simulink library "myLibrary"  (R2023b)
settings: Solver=VariableStepAuto  StartTime=0.0  StopTime=10.0  RelTol=1e-3
undefined symbols (not defined in the file): Cac_n1, ctrl1, Da, delta_slk, Discrete, dtha, ee_sli_rtmsupport, FA, gcbh, Ha, Ini, init_DCline, init_IPC, init_line, init_load, init_SG, init_shunt, init_TH, init_trafo, init_user, init_VSC, initMachineBlocks, Ka, Lf, Llkd_pu, Llkq1_pu, magnitude, NET, P, plots_step, q0, Rac_n1, Radd, Rkd_pu, Rkq1_pu, Rload_add, sim_config, sps_rtmsupport, spsSteamTurbineModel, T_DC_NET, T_global, T_IPC, T_load, T_NET, T_SG, T_shunt, T_STATCOM, T_TH, T_trafo, T_user, T_VSC, Ts, tstep, Udiff_a, V1
libraries: spsSeriesRLCBranchLib x120, eeGeneralControl x83, $bdroot x78, spsCurrentMeasurementLib x53, spsParallelRLCBranchLib x39, spsVoltageMeasurementLib x37, spsControlledVoltageSourceLib x30, simulink x29, spsFirstOrderFilterLib x18, spsMeasurementModel x13, spsThreePhaseVIMeasurementLib x5, dspsigops x4
(part 5 of 16)

== system myLibrary/WT ==
  Constant1 : Constant  Value=[ 2/3 1/3; -1/3 1/3 ; -1/3 -2/3]
  Constant5 : Constant  Value=[ 2/3 1/3; -1/3 1/3 ; -1/3 -2/3]
  Control : Subsystem
      settings: PortSchema="{\"entries\":[{\"content\":{\"sides\":[{\"content\":{},\"type\":\"ConnectorPlacement.EquallySpacedRectSide\",\"uuid\":\"681c0b5f-022d-4b6d-8fe2-73940743a76e\"},{\"content\":{\"side\":\"RIGHT\"},\"type\":\"ConnectorPlacement.EquallySpacedRectSide\",\"uuid\":\"e9b400c8-e13f-4caf-91a1-f348979675fd\"},{\"content\":{\"connectorIds\":[\"In1\",\"Out1\",\"Out2\"],\"side\":\"TOP\"},\"type\":\"ConnectorPlacement.EquallySpacedRectSide\",\"uuid\":\"348007cb-ce67-4c45-ad7b-36ba89db6185\"},{\"content\":{\"connectorIds\":[\"In2\",\"In3\",\"In4\",\"In5\"],\"side\":\"BOTTOM\"},\"type\":\"ConnectorPlacement.EquallySpacedRectSide\",\"uuid\":\"fd6a847a-5d69-44cd-a0d1-495126761350\"}]},\"type\":\"ConnectorPlacement.EquallySpacedConnector\",\"uuid\":\"d16b8cae-5ced-4c76-a87e-983e154fb48f\"}],\"packageUris\":[\"http://schema.mathworks.com/mf0/Connector/R2020b\"],\"version\":\"1.0\"}"
  Current Measurement20 : spsCurrentMeasurementLib/Current Measurement  PhasorSimulation=off  OutputType=Complex  PSBequivalent=0
  Current Measurement21 : spsCurrentMeasurementLib/Current Measurement  PhasorSimulation=off  OutputType=Complex  PSBequivalent=0
  Current Measurement25 : spsCurrentMeasurementLib/Current Measurement  PhasorSimulation=off  OutputType=Complex  PSBequivalent=0
  Delay : Subsystem
  Electrical : Subsystem
  Filter Ig : Subsystem
  Filter Is : Subsystem
  Filter U : Subsystem
  Filter Vdc : Subsystem
  Filter Vg : Subsystem
  Gain : Gain  Gain=sqrt(2)/sqrt(3)
  Ig_l2g : Gain  Gain=1/T_VSC.Sbpu_l2g
  Ig_l2g1 : Gain  Gain=sqrt(3/2)
  Ig_l2g2 : Gain  Gain=sqrt(3/2)
  Is_l2g : Gain  Gain=1/T_VSC.Sbpu_l2g
  Mux1 : Mux  Inputs=2
  Mux10 : Mux  Inputs=2
  Mux4 : Mux  Inputs=3
  Product1 : Product  Multiplication=Matrix(*)
  Product4 : Product  Multiplication=Matrix(*)
  Series RLC Branch1 : spsSeriesRLCBranchLib/Series RLC Branch  LConnTagsString=__new0  RConnTagsString=__new0  BranchType=RL  Resistance=initVSC.Rtr  Inductance=initVSC.Ltr  SetiL0=off  InitialCurrent=initVSC.Iga  Capacitance=P.C  Setx0=on  InitialVoltage=P.C  Measurements=None
  Series RLC Branch10 : spsSeriesRLCBranchLib/Series RLC Branch  LConnTagsString=__new0  RConnTagsString=__new0  BranchType=R  Resistance=initVSC.Rac  Inductance=Lf  SetiL0=off  InitialCurrent=0  Capacitance=Cac_n1  Setx0=on  InitialVoltage=vcini_n1  Measurements=None
  Series RLC Branch2 : spsSeriesRLCBranchLib/Series RLC Branch  LConnTagsString=__new0  RConnTagsString=__new0  BranchType=RL  Resistance=initVSC.Rtr  Inductance=initVSC.Ltr  SetiL0=on  InitialCurrent=initVSC.Igb  Capacitance=P.C  Setx0=on  InitialVoltage=P.C  Measurements=None
  Series RLC Branch3 : spsSeriesRLCBranchLib/Series RLC Branch  LConnTagsString=__new0  RConnTagsString=__new0  BranchType=RL  Resistance=initVSC.Rtr  Inductance=initVSC.Ltr  SetiL0=on  InitialCurrent=initVSC.Igc  Capacitance=P.C  Setx0=on  InitialVoltage=P.C  Measurements=None
  Series RLC Branch4 : spsSeriesRLCBranchLib/Series RLC Branch  LConnTagsString=__new0  RConnTagsString=__new0  BranchType=C  Resistance=Rac_n1  Inductance=Lf  SetiL0=off  InitialCurrent=0  Capacitance=initVSC.Cac  Setx0=on  InitialVoltage=initVSC.Ucap_b  Measurements=None
  Series RLC Branch5 : spsSeriesRLCBranchLib/Series RLC Branch  LConnTagsString=__new0  RConnTagsString=__new0  BranchType=C  Resistance=Rac_n1  Inductance=Lf  SetiL0=off  InitialCurrent=0  Capacitance=initVSC.Cac  Setx0=on  InitialVoltage=initVSC.Ucap_a  Measurements=None
  Series RLC Branch6 : spsSeriesRLCBranchLib/Series RLC Branch  LConnTagsString=__new0  RConnTagsString=__new0  BranchType=R  Resistance=initVSC.Rac  Inductance=Lf  SetiL0=off  InitialCurrent=0  Capacitance=Cac_n1  Setx0=on  InitialVoltage=vcini_n1  Measurements=None
  Series RLC Branch8 : spsSeriesRLCBranchLib/Series RLC Branch  LConnTagsString=__new0  RConnTagsString=__new0  BranchType=R  Resistance=initVSC.Rac  Inductance=Lf  SetiL0=off  InitialCurrent=0  Capacitance=Cac_n1  Setx0=on  InitialVoltage=vcini_n1  Measurements=None
  Series RLC Branch9 : spsSeriesRLCBranchLib/Series RLC Branch  LConnTagsString=__new0  RConnTagsString=__new0  BranchType=C  Resistance=Rac_n1  Inductance=Lf  SetiL0=off  InitialCurrent=0  Capacitance=initVSC.Cac  Setx0=on  InitialVoltage=initVSC.Ucap_c  Measurements=None
  U_g2l : Gain  Gain=sqrt(3)/sqrt(2)
  U_g2l1 : Gain  Gain=sqrt(3)/sqrt(2)
  Voltage Measurement{,1,5..6} (4 alike) : spsVoltageMeasurementLib/Voltage Measurement  PhasorSimulation=off  OutputType=Complex  PSBequivalent=0
  VA : PMIOPort  Side=Right
  VB : PMIOPort  Port=2  Side=Right
  VC : PMIOPort  Port=3  Side=Right
  wires:
  Voltage Measurement1/1 -> Mux10/2
  Constant5/1 -> Product4/1
  Mux10/1 -> Product4/2
  Voltage Measurement/1 -> Mux10/1
  Is_l2g/1 -> Ig_l2g2/1
  U_g2l/1 -> Control/2(U)
  Current Measurement20/1 -> Mux4/2
  Current Measurement21/1 -> Mux4/1
  Current Measurement25/1 -> Mux4/3
  Ig_l2g/1 -> Control/1(ig_abc)
  Control/2(Pac) -> Electrical/1(Pac)
  Voltage Measurement6/1 -> Mux1/2
  Constant1/1 -> Product1/1
  Voltage Measurement5/1 -> Mux1/1
  Mux1/1 -> Product1/2
  U_g2l1/1 -> Control/3(Vg)
  Ig_l2g1/1 -> Ig_l2g/1
  Ig_l2g2/1 -> Control/4(Iss)
  Control/1(Vdiff_abc) -> Gain/1
  Filter Ig/1(Out1) -> Ig_l2g1/1
  Mux4/1 -> Filter Ig/1(In1)
  Filter Vg/1(Out1) -> U_g2l1/1
  Product1/1 -> Filter Vg/1(In1)
  Filter U/1(Out1) -> U_g2l/1
  Product4/1 -> Filter U/1(In1)
  Electrical/1(Vdc) -> Filter Vdc/1(In1)
  Filter Vdc/1(Out1) -> Control/5(Vdc)
  Filter Is/1(Out1) -> Is_l2g/1
  Electrical/2(Is) -> Filter Is/1(In1)
  Delay/1(Out1) -> Electrical/2(vdiff)
  Gain/1 -> Delay/1(In1)
  connections:
  VB/RConn1 -- Current Measurement20/RConn1
  Series RLC Branch1/LConn1 -- Series RLC Branch5/LConn1 -- Voltage Measurement/LConn1 -- Electrical/LConn1
  Voltage Measurement1/LConn2 -- Series RLC Branch9/LConn1 -- Series RLC Branch3/LConn1 -- Electrical/LConn3
  VA/RConn1 -- Current Measurement21/RConn1
  Voltage Measurement1/LConn1 -- Voltage Measurement/LConn2 -- Series RLC Branch4/LConn1 -- Series RLC Branch2/LConn1 -- Electrical/LConn2
  Current Measurement25/RConn1 -- VC/RConn1
  Series RLC Branch1/RConn1 -- Voltage Measurement5/LConn1 -- Current Measurement21/LConn1
  Series RLC Branch2/RConn1 -- Voltage Measurement6/LConn1 -- Voltage Measurement5/LConn2 -- Current Measurement20/LConn1
  Series RLC Branch3/RConn1 -- Voltage Measurement6/LConn2 -- Current Measurement25/LConn1
  Series RLC Branch6/LConn1 -- Series RLC Branch5/RConn1
  Series RLC Branch4/RConn1 -- Series RLC Branch8/LConn1
  Series RLC Branch10/LConn1 -- Series RLC Branch9/RConn1
  Series RLC Branch10/RConn1 -- Series RLC Branch8/RConn1 -- Series RLC Branch6/RConn1

== system myLibrary/qd transform ==
  abc : Inport
  angle : Inport  Port=2
  Demux8 : Demux  Outputs=3
  qd0 Transformation : Subsystem
  q : Outport
  d : Outport  Port=2
  wires:
  qd0 Transformation/1(q) -> q/1  "q"
  Demux8/1 -> qd0 Transformation/1(a)
  qd0 Transformation/2(d) -> d/1  "d"
  Demux8/2 -> qd0 Transformation/2(b)
  abc/1 -> Demux8/1
  Demux8/3 -> qd0 Transformation/3(c)
  angle/1 -> qd0 Transformation/4(Angle)

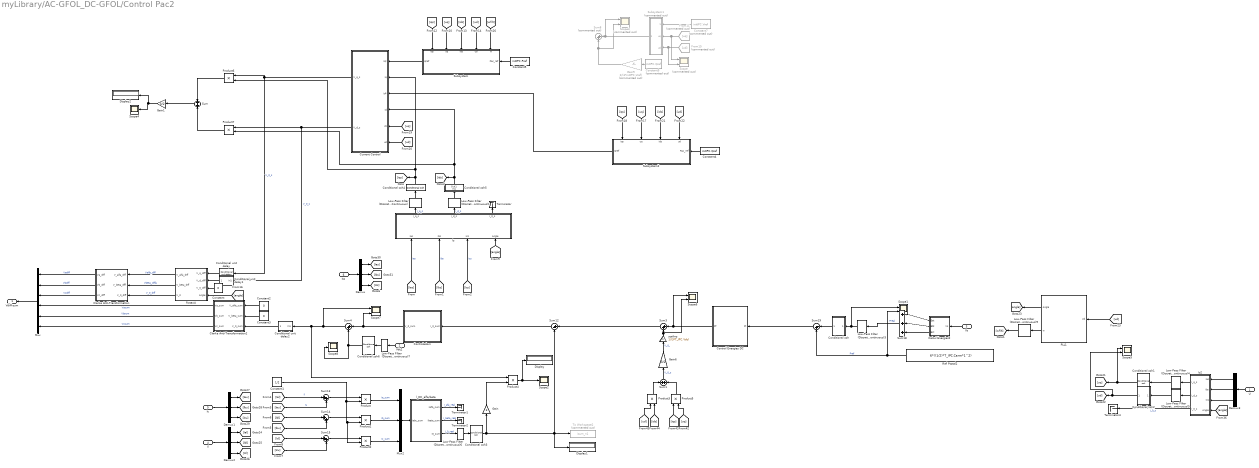
== system myLibrary/AC-GFOL_DC-GFOL/Control Pac2 ==
  U : Inport
  Vdc2 : Inport  Port=2
  Vs : Inport  Port=3
  Il : Inport  Port=4
  Iu : Inport  Port=5
  Iss : Inport  Port=6
  Calcul Energies2 : Subsystem
  Clarke Anti-Transformation : Subsystem
  Clarke Anti-Transformation2 : Subsystem
  Conditional unit delay : $bdroot/GFOL/Control/Conditional unit delay  SystemSampleTime=-1  VariantActivationTime=update diagram  AllowFlexibleInterface=on  Latency=0  AutoFrameSizeCalculation=off
      link override Constant4: Value=T_IPC.tau_cmd
      link override Unit Delay2: InitialCondition=initIPC.vdiffq  SampleTime=T_IPC.tau_cmd
  Conditional unit delay1 : Subsystem
  Conditional unit delay2 : Subsystem
  Conditional zoh : Subsystem
  Conditional zoh{1,3..4,6} (4 alike) : $bdroot/AC-GFOL_DC-GFOL/Control Pac2/Conditional zoh  SystemSampleTime=-1  VariantActivationTime=update diagram  AllowFlexibleInterface=on  Latency=0  AutoFrameSizeCalculation=off
  Conditional zoh2 : Subsystem
  Conditional zoh5 : Subsystem
  Constant : Constant  Value=0
  Constant1 : Constant  Value=1/2
  Constant2 : Constant  Value=0
  Constant3 : Constant  Value=0
  Constant4 : Constant  Value=initIPC.Qref
  Constant5 : Constant  Value=initIPC.Pref
  Constant7 : Constant  Commented=on  Value=initIPC.Vref
  Constant9 : Constant  Commented=on  Value=initIPC.Qref
  Control Energies DC : Subsystem
  Controladors : Subsystem
  Current Control : Subsystem
  Demux{,1..3} (4 alike) : Demux  Outputs=3
  Display : Display
  Display1 : Display
  Display2 : Display
  From11 : From  Commented=on  GotoTag=uq
  From15 : From  Commented=on  GotoTag=ud
  Gain : Gain  Gain=3
  Gain1 : Gain  Gain=3/2
  Gain6 : Gain  Gain=3/2
  Gain9 : Gain  Commented=on  Gain=2/(3*initIPC.Vref)
  Is : Subsystem
  Is2 : Subsystem
  Low-Pass Filter (Discrete or Continuous) : eeGeneralControl/Low-Pass Filter (Discrete or Continuous)  K=1  T=T_IPC.delay  B=inf  A=-inf  init_option=Specify as parameter  x0=initIPC.idiffq  Ts=0
  Low-Pass Filter (Discrete or Continuous)1 : eeGeneralControl/Low-Pass Filter (Discrete or Continuous)  K=1  T=T_IPC.delay  B=inf  A=-inf  init_option=Specify as parameter  x0=initIPC.idiffd  Ts=0
  Low-Pass Filter (Discrete or Continuous)3 : eeGeneralControl/Low-Pass Filter (Discrete or Continuous)  K=1  T=T_IPC.delay  B=inf  A=-inf  init_option=Specify as parameter  x0=6*((1/2)*T_IPC.Carm*1^2)  Ts=0
  Low-Pass Filter (Discrete or Continuous)4 : eeGeneralControl/Low-Pass Filter (Discrete or Continuous)  K=1  T=T_IPC.delay  B=inf  A=-inf  init_option=Specify as parameter  x0=initIPC.uq  Ts=0
  Low-Pass Filter (Discrete or Continuous)5 : eeGeneralControl/Low-Pass Filter (Discrete or Continuous)  K=1  T=T_IPC.delay  B=inf  A=-inf  init_option=Specify as parameter  x0=initIPC.ud  Ts=0
  Low-Pass Filter (Discrete or Continuous)6 : eeGeneralControl/Low-Pass Filter (Discrete or Continuous)  K=1  T=T_IPC.delay  B=inf  A=-inf  init_option=Specify as parameter  x0=initIPC.isum0_DC  Ts=0
  Low-Pass Filter (Discrete or Continuous)7 : eeGeneralControl/Low-Pass Filter (Discrete or Continuous)  K=1  T=T_IPC.delay  B=inf  A=-inf  init_option=Specify as parameter  x0=initIPC.Vdc  Ts=0
  Low-Pass Filter (Discrete or Continuous)9 : eeGeneralControl/Low-Pass Filter (Discrete or Continuous)  K=1  T=T_IPC.tw  B=inf  A=-inf  init_option=Specify as parameter  x0=2*pi*T_IPC.fb  Ts=0
  Mux : Mux  Inputs=6
  Mux2 : Mux  Inputs=3
  PLL1 : Subsystem
  Product{,1..7} (8 alike) : Product
  Ref Ptotal2 : Constant  Value=6*((1/2)*T_IPC.Carm*1^2)
  Rotació : Subsystem
  Scope : Scope  Commented=on  NumInputPorts=2
  Scope{1,5..7} (4 alike) : Scope  NumInputPorts=2
  Scope2 : Scope
  Scope3 : Scope  Commented=on  NumInputPorts=2
  Scope4 : Scope
  Scope8 : Scope
  Subsystem : Subsystem
      settings: PortSchema="{\"entries\":[{\"content\":{\"sides\":[{\"content\":{\"connectorIds\":[\"Out1\"]},\"type\":\"ConnectorPlacement.EquallySpacedRectSide\",\"uuid\":\"dea8424c-00e8-4bd8-a696-176e9d81b4b0\"},{\"content\":{\"connectorIds\":[\"In6\"],\"side\":\"RIGHT\"},\"type\":\"ConnectorPlacement.EquallySpacedRectSide\",\"uuid\":\"15b830a2-0897-480b-96a6-ff349e082a47\"},{\"content\":{\"connectorIds\":[\"In1\",\"In2\",\"In3\",\"In4\",\"In5\"],\"side\":\"TOP\"},\"type\":\"ConnectorPlacement.EquallySpacedRectSide\",\"uuid\":\"07916eec-e3fd-4ba3-9129-5b3a9aa06051\"}]},\"type\":\"ConnectorPlacement.EquallySpacedConnector\",\"uuid\":\"22000632-3c2a-414c-a4d7-471046f1c1a1\"}],\"packageUris\":[\"http://schema.mathworks.com/mf0/Connector/R2020b\"],\"version\":\"1.0\"}"
  Subsystem1 : Subsystem  Commented=on
      settings: PortSchema="{\"entries\":[{\"content\":{\"sides\":[{\"content\":{\"connectorIds\":[\"Out1\"]},\"type\":\"ConnectorPlacement.EquallySpacedRectSide\",\"uuid\":\"effe47ce-951a-4fb1-8fc1-e963775b8c82\"},{\"content\":{\"connectorIds\":[\"In1\",\"In2\",\"In3\"],\"side\":\"RIGHT\"},\"type\":\"ConnectorPlacement.EquallySpacedRectSide\",\"uuid\":\"a859b59d-6664-4e67-878a-4ecbefd8f8f0\"},{\"content\":{\"connectorIds\":[],\"side\":\"TOP\"},\"type\":\"ConnectorPlacement.EquallySpacedRectSide\",\"uuid\":\"0b762440-c8d9-40a7-a5db-13c46bc0406e\"}]},\"type\":\"ConnectorPlacement.EquallySpacedConnector\",\"uuid\":\"dbc4fef9-6b40-4568-97c6-19f27935f422\"}],\"packageUris\":[\"http://schema.mathworks.com/mf0/Connector/R2020b\"],\"version\":\"1.0\"}"
  Subsystem2 : Subsystem
      settings: PortSchema="{\"entries\":[{\"content\":{\"sides\":[{\"content\":{\"connectorIds\":[\"Out1\"]},\"type\":\"ConnectorPlacement.EquallySpacedRectSide\",\"uuid\":\"dea8424c-00e8-4bd8-a696-176e9d81b4b0\"},{\"content\":{\"connectorIds\":[\"In5\"],\"side\":\"RIGHT\"},\"type\":\"ConnectorPlacement.EquallySpacedRectSide\",\"uuid\":\"15b830a2-0897-480b-96a6-ff349e082a47\"},{\"content\":{\"connectorIds\":[\"In1\",\"In2\",\"In3\",\"In4\"],\"side\":\"TOP\"},\"type\":\"ConnectorPlacement.EquallySpacedRectSide\",\"uuid\":\"07916eec-e3fd-4ba3-9129-5b3a9aa06051\"}]},\"type\":\"ConnectorPlacement.EquallySpacedConnector\",\"uuid\":\"22000632-3c2a-414c-a4d7-471046f1c1a1\"}],\"packageUris\":[\"http://schema.mathworks.com/mf0/Connector/R2020b\"],\"version\":\"1.0\"}"
  Sum : Sum
  Sum1 : Sum
  Sum12 : Sum  Inputs=|+-
  Sum{3..4,13..15} (5 alike) : Sum  Inputs=|++
  Sum18 : Sum  Inputs=|+++
  Sum19 : Sum  Inputs=|-+
  Sum8 : Sum  Commented=on  Inputs=|++
  Terminator{,1..2,4} (4 alike) : Terminator
  To Workspace2 : ToWorkspace  Commented=on  VariableName=isum_n1  SampleTime=plots_step
  l_DC_alfa/beta : Subsystem
  scaling : Gain  Gain=1/(3*T_IPC.Vdc)
  Vdiff-sum : Outport
  wires:
  [wfilt] -> Subsystem/5(w)
  Low-Pass Filter (Discrete or Continuous)9/1 -> [wfilt]
  PLL1/2(w) -> Low-Pass Filter (Discrete or Continuous)9/1
  Low-Pass Filter (Discrete or Continuous)6/1 -> Conditional zoh3/1
  Is/3(I_0_s) -> Terminator/1
  Low-Pass Filter (Discrete or Continuous)7/1 -> Conditional zoh6/1
  Low-Pass Filter (Discrete or Continuous)5/1 -> Conditional zoh2/1(In1)
  Low-Pass Filter (Discrete or Continuous)1/1 -> Conditional zoh5/1(In1)
  Low-Pass Filter (Discrete or Continuous)/1 -> Conditional zoh4/1
  Ref Ptotal2/1 -> Sum19/2, Scope1/2  "Pref"
  Calcul Energies2/1(Eat) -> Sum18/1
  Constant2/1 -> Clarke Anti-Transformation2/1(V_alfa_sum)
  Constant3/1 -> Clarke Anti-Transformation2/2(V_beta_sum)
  Mux/1 -> Vdiff-sum/1
  Clarke Anti-Transformation2/1(Va_sum) -> Mux/4  "Vasum"
  Clarke Anti-Transformation2/2(Vb_sum) -> Mux/5  "Vbsum"
  Clarke Anti-Transformation/3(Vc_diff) -> Mux/3  "Vcdiff"
  Clarke Anti-Transformation/2(Vb_diff) -> Mux/2  "Vbdiff"
  Clarke Anti-Transformation/1(Va_diff) -> Mux/1  "Vadiff"
  Rotació/1(V_alfa_diff) -> Clarke Anti-Transformation/1(V_alfa_diff)  "Valfa_diff"
  Rotació/3(V_0) -> Clarke Anti-Transformation/3(V_0_diff)  "V_0_diff"
  [Ias] -> Is/1(Ias)  "Ias"
  [Ics] -> Is/3(Ics)  "Ics"
  [Ibs] -> Is/2(Ibs)  "Ibs"
  Rotació/2(V_beta_diff) -> Clarke Anti-Transformation/2(V_beta_dfff)  "Vbeta_diffa"
  Mux2/1 -> l_DC_alfa/beta/1(Iabc_sum)
  Product/1 -> Mux2/1  "Ia_sum"
  [Ial] -> Sum13/1  "Il"
  [Iau] -> Sum13/2  "Iu"
  Sum13/1 -> Product/1
  Constant1/1 -> Product2/2, Product1/2, Product/2
  Product1/1 -> Mux2/2  "Ib_sum"
  [Ibl] -> Sum14/1
  [Ibu] -> Sum14/2
  Sum14/1 -> Product1/1
  Product2/1 -> Mux2/3  "Ic_sum"
  [Icl] -> Sum15/1
  [Icu] -> Sum15/2
  Sum15/1 -> Product2/1
  Clarke Anti-Transformation2/3(Vc_sum) -> Mux/6  "Vcsum"
  Iu/1 -> Demux1/1
  Demux2/2 -> [Ibl]
  Demux1/1 -> [Iau]
  Demux1/3 -> [Icu]
  Il/1 -> Demux2/1
  Demux2/3 -> [Icl]
  Demux2/1 -> [Ial]
  Demux1/2 -> [Ibu]
  Demux3/2 -> Is2/2(Ibs)
  [angle] -> Is2/4(Angle)
  PLL1/1(Angle) -> [angle]
  [ud] -> PLL1/1(Ud)
  U/1 -> Demux3/1
  Demux3/3 -> Is2/3(Ics)
  Demux3/1 -> Is2/1(Ias)
  Demux/1 -> [Ias]
  Demux/2 -> [Ibs]
  Demux/3 -> [Ics]
  Iss/1 -> Demux/1
  Vs/1 -> Calcul Energies2/1(Vs)
  Calcul Energies2/3(Ect) -> Sum18/3
  Calcul Energies2/2(Ebt) -> Sum18/2
  [angle] -> Is/4(Angle)
  [angle] -> Rotació/4(Angle)
  Current Control/1(V_q_s) -> Product6/1, Conditional unit delay/1  "V_0_s"
  [uq] -> Current Control/5(uq)
  [ud] -> Current Control/6(ud)
  Controladors/1(V_0_sum) -> Scope7/2, Sum4/1
  Sum12/1 -> Controladors/1(I_0_sum)
  Sum19/1 -> Control Energies DC/1(Pt)
  [uq] -> Subsystem/2(uq)
  [iqs] -> Subsystem/1(iqs)
  [ud] -> Subsystem/4(ud)
  [ids] -> Subsystem/3(ids)
  Constant7/1 -> Subsystem1/1(uref)
  From11/1 -> Scope/1, Subsystem1/2(uq)
  From15/1 -> Scope/2, Subsystem1/3(ud)
  Is2/3(I_0_s) -> Terminator4/1  "I_0_s"
  Constant5/1 -> Subsystem/6(Pac_ref)
  Subsystem/1(iqref) -> Current Control/1(Iq*)
  [ud] -> Product3/1
  [uq] -> Product5/2
  Gain6/1 -> scaling/1  "V_0_"
  Sum1/1 -> Gain6/1  "V_0_s"
  Product5/1 -> Sum1/2
  Control Energies DC/1(Pt') -> Scope6/1, Sum3/1
  [iqs] -> Product5/1
  scaling/1 -> Scope6/2, Sum3/2
  Sum3/1 -> Sum12/1
  Product3/1 -> Sum1/1
  [ids] -> Product3/2
  Subsystem1/1(idref) -> Scope3/1, Sum8/1
  Constant9/1 -> Gain9/1
  Gain9/1 -> Scope3/2, Sum8/2
  Current Control/2(V_d_s) -> Product7/1, Conditional unit delay1/1(In1)  "V_0_s"
  Constant/1 -> Rotació/3(V_0_diff)
  l_DC_alfa/beta/1(Ialfa_sum) -> Terminator1/1  "I_afa_real"
  l_DC_alfa/beta/2(Ibeta_sum) -> Terminator2/1  "I_beta_real"
  Product4/1 -> Display/1, Scope2/1
  Gain/1 -> Product4/2
  Sum/1 -> Gain1/1
  Product6/1 -> Sum/1
  Product7/1 -> Sum/2
  Gain1/1 -> Display2/1, Scope4/1
  Constant4/1 -> Subsystem2/5(Pac_ref)
  [ids] -> Subsystem2/3(ids)
  [ud] -> Subsystem2/4(ud)
  [iqs] -> Subsystem2/1(iqs)
  [uq] -> Subsystem2/2(uq)
  Subsystem2/1(iqref) -> Current Control/3(Id*)
  Sum4/1 -> Scope7/1, Product4/1, Conditional unit delay2/1(In1)
  Conditional unit delay/1 -> Rotació/1(V_q_diff)
  Conditional unit delay1/1(Out1) -> Rotació/2(V_d_diff)
  Conditional unit delay2/1(Out1) -> Clarke Anti-Transformation2/3(V_0_sum)
  Is/1(I_q_s) -> Low-Pass Filter (Discrete or Continuous)/1  "I_q_s"
  Conditional zoh4/1 -> Product6/2, Current Control/2(Iq), [iqs]
  Is/2(I_d_s) -> Low-Pass Filter (Discrete or Continuous)1/1  "I_d_s"
  Conditional zoh5/1(Out1) -> Product7/2, Current Control/4(Id), [ids]
  Vdc2/1 -> Low-Pass Filter (Discrete or Continuous)7/1
  Conditional zoh6/1 -> Sum4/2, Scope8/1
  l_DC_alfa/beta/3(I0_sum) -> Low-Pass Filter (Discrete or Continuous)6/1  "I_0_real"
  Conditional zoh3/1 -> Gain/1, Display1/1, To Workspace2/1, Sum12/2
  Conditional zoh/1(Out1) -> Sum19/1
  Low-Pass Filter (Discrete or Continuous)3/1 -> Scope1/1, Conditional zoh/1(In1)
  Sum18/1 -> Low-Pass Filter (Discrete or Continuous)3/1  "Preal"
  Is2/1(I_q_s) -> Low-Pass Filter (Discrete or Continuous)4/1
  Low-Pass Filter (Discrete or Continuous)4/1 -> Conditional zoh1/1
  Conditional zoh1/1 -> Scope5/1, [uq]
  Conditional zoh2/1(Out1) -> Scope5/2, [ud]
  Is2/2(I_d_s) -> Low-Pass Filter (Discrete or Continuous)5/1

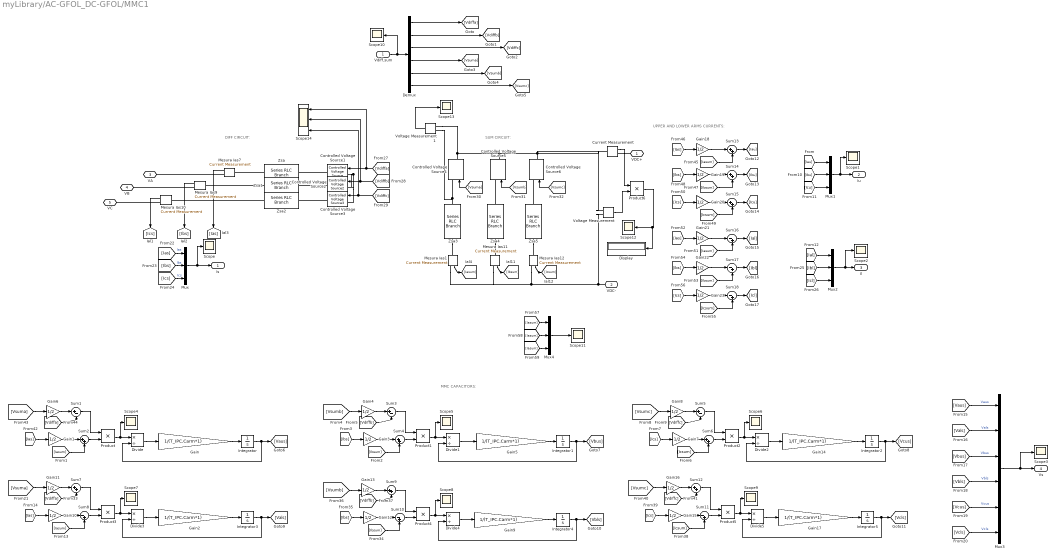
== system myLibrary/AC-GFOL_DC-GFOL/MMC1 ==
  note: UPPER AND LOWER ARMS CURRENTS:
  note: MMC CAPACITORS:
  note: SUM CIRCUIT:
  note: DIFF CIRCUIT:
  Vdiff,sum : Inport
  Controlled Voltage Source1 : spsControlledVoltageSourceLib/Controlled Voltage Source  Initialize=on  Source_Type=AC  Amplitude=initIPC.Udiff_mag  Phase=initIPC.angle_vdiff  Frequency=T_IPC.fb  Measurements=None
  Controlled Voltage Source2 : $bdroot/AC-GFOL_DC-GFOR/MMC1/Controlled Voltage Source2  Initialize=on  Source_Type=AC  Amplitude=initIPC.Udiff_mag  Phase=initIPC.angle_vdiff-120  Frequency=T_IPC.fb  Measurements=None
      settings: LibrarySourceBlock=spsControlledVoltageSourceLib/Controlled Voltage Source
  Controlled Voltage Source3 : $bdroot/AC-GFOL_DC-GFOR/MMC1/Controlled Voltage Source3  Initialize=on  Source_Type=AC  Amplitude=initIPC.Udiff_mag  Phase=initIPC.angle_vdiff+120  Frequency=T_IPC.fb  Measurements=None
      settings: LibrarySourceBlock=spsControlledVoltageSourceLib/Controlled Voltage Source
  Controlled Voltage Source4 : spsControlledVoltageSourceLib/Controlled Voltage Source  Initialize=on  Source_Type=DC  Amplitude=initIPC.Usuma  Phase=0  Frequency=0  Measurements=None
  Controlled Voltage Source5 : spsControlledVoltageSourceLib/Controlled Voltage Source  Initialize=on  Source_Type=DC  Amplitude=initIPC.Usumb  Phase=angle(Udiff_a)*180/pi  Frequency=60  Measurements=None
  Controlled Voltage Source6 : spsControlledVoltageSourceLib/Controlled Voltage Source  Initialize=on  Source_Type=DC  Amplitude=initIPC.Usumc  Phase=angle(Udiff_a)*180/pi  Frequency=60  Measurements=None
  Current Measurement : spsCurrentMeasurementLib/Current Measurement  PhasorSimulation=off  OutputType=Complex  PSBequivalent=0
  Demux : Demux  Outputs=6
  Display : Display
  Divide{,1..5} (6 alike) : Product  Inputs=*/
  Gain{,2,5,9,14,17} (6 alike) : Gain  Gain=1/(T_IPC.Carm*1)
  Gain{1,3..4,6..8,10..13,15..16,18..23} (18 alike) : Gain  Gain=1/2
  Integrator{,1..5} (6 alike) : Integrator  InitialCondition=1
  Mesura Ias{1,7,9..12} (6 alike) : spsCurrentMeasurementLib/Current Measurement  PhasorSimulation=off  OutputType=Complex  PSBequivalent=0
  Mux{,1..2,4} (4 alike) : Mux  Inputs=3
  Mux3 : Mux  Inputs=6
  Product{,1..6} (7 alike) : Product
  Scope{,1..13} (14 alike) : Scope
  Scope14 : Scope  NumInputPorts=3
  Sum1 : Sum  Inputs=|+-
  Sum{8,10..11,16..18} (6 alike) : Sum  Inputs=|-+
  Sum{2,4,6..7,9,12..15} (9 alike) : Sum  Inputs=|++
  Sum3 : Sum  Inputs=|+-
  Sum5 : Sum  Inputs=|+-
  Voltage Measurement : spsVoltageMeasurementLib/Voltage Measurement  PhasorSimulation=off  OutputType=Complex  PSBequivalent=0
  Voltage Measurement1 : spsVoltageMeasurementLib/Voltage Measurement  PhasorSimulation=off  OutputType=Complex  PSBequivalent=0
  Zsa : spsSeriesRLCBranchLib/Series RLC Branch  LConnTagsString=__new0  RConnTagsString=__new0  BranchType=RL  Resistance=(T_IPC.Rc+T_IPC.Ra/2)/T_IPC.Sbpu_l2g  Inductance=(T_IPC.Lc+T_IPC.La/2)/T_IPC.Sbpu_l2g  SetiL0=on  InitialCurrent=initIPC.Isa*T_IPC.Sbpu_l2g  Capacitance=1e-6  Setx0=off  InitialVoltage=0  Measurements=None
  Zsa1 : spsSeriesRLCBranchLib/Series RLC Branch  LConnTagsString=__new0  RConnTagsString=__new0  BranchType=RL  Resistance=(T_IPC.Rc+T_IPC.Ra/2)/T_IPC.Sbpu_l2g  Inductance=(T_IPC.Lc+T_IPC.La/2)/T_IPC.Sbpu_l2g  SetiL0=on  InitialCurrent=initIPC.Isb*T_IPC.Sbpu_l2g  Capacitance=1e-6  Setx0=off  InitialVoltage=0  Measurements=None
  Zsa2 : spsSeriesRLCBranchLib/Series RLC Branch  LConnTagsString=__new0  RConnTagsString=__new0  BranchType=RL  Resistance=(T_IPC.Rc+T_IPC.Ra/2)/T_IPC.Sbpu_l2g  Inductance=(T_IPC.Lc+T_IPC.La/2)/T_IPC.Sbpu_l2g  SetiL0=on  InitialCurrent=initIPC.Isc*T_IPC.Sbpu_l2g  Capacitance=1e-6  Setx0=off  InitialVoltage=0  Measurements=None
  Zsa3 : spsSeriesRLCBranchLib/Series RLC Branch  LConnTagsString=__new0  RConnTagsString=__new0  BranchType=RL  Resistance=(2*T_IPC.Ra)/T_IPC.Sbpu_l2g  Inductance=(2*T_IPC.La)/T_IPC.Sbpu_l2g  SetiL0=on  InitialCurrent=initIPC.isum0_DC*T_IPC.Sbpu_l2g  Capacitance=1e-6  Setx0=off  InitialVoltage=0  Measurements=None
  Zsa4 : spsSeriesRLCBranchLib/Series RLC Branch  LConnTagsString=__new0  RConnTagsString=__new0  BranchType=RL  Resistance=(2*T_IPC.Ra)/T_IPC.Sbpu_l2g  Inductance=(2*T_IPC.La)/T_IPC.Sbpu_l2g  SetiL0=on  InitialCurrent=initIPC.isum0_DC*T_IPC.Sbpu_l2g  Capacitance=1e-6  Setx0=off  InitialVoltage=0  Measurements=None
  Zsa5 : spsSeriesRLCBranchLib/Series RLC Branch  LConnTagsString=__new0  RConnTagsString=__new0  BranchType=RL  Resistance=(2*T_IPC.Ra)/T_IPC.Sbpu_l2g  Inductance=(2*T_IPC.La)/T_IPC.Sbpu_l2g  SetiL0=on  InitialCurrent=initIPC.isum0_DC*T_IPC.Sbpu_l2g  Capacitance=1e-6  Setx0=off  InitialVoltage=0  Measurements=None
  VDC+ : PMIOPort  Side=Right
  VDC- : PMIOPort  Port=2  Side=Right
  VA : PMIOPort  Port=3  Side=Left
  VB : PMIOPort  Port=4  Side=Left
  VC : PMIOPort  Port=5  Side=Left
  Is : Outport
  Iu : Outport  Port=2
  Il : Outport  Port=3
  Vs : Outport  Port=4
  wires:
  [Ibl] -> Mux2/2
  Sum18/1 -> [Icl]
  Gain23/1 -> Sum18/1
  [Ics] -> Gain23/1
  [Icsum] -> Sum18/2
  [Ibsum] -> Sum17/2
  [Ibs] -> Gain22/1
  Gain22/1 -> Sum17/1
  Sum17/1 -> [Ibl]
  Sum16/1 -> [Ial]
  Gain21/1 -> Sum16/1
  [Ias] -> Gain21/1
  [Iasum] -> Sum16/2
  Sum15/1 -> [Icu]
  [Icsum] -> Sum15/2
  Gain20/1 -> Sum15/1
  [Ics] -> Gain20/1
  [Ibs] -> Gain19/1
  Gain19/1 -> Sum14/1
  [Ibsum] -> Sum14/2
  Sum14/1 -> [Ibu]
  Sum13/1 -> [Iau]
  [Iasum] -> Sum13/2
  Gain18/1 -> Sum13/1
  [Ias] -> Gain18/1
  Sum11/1 -> Product5/2
  Product5/1 -> Scope9/1, Divide5/1
  Divide5/1 -> Gain17/1
  Gain17/1 -> Integrator5/1
  Integrator5/1 -> [Vcls], Divide5/2
  Gain16/1 -> Sum12/1
  [Vdiffc] -> Sum12/2
  [Icsum] -> Sum11/2
  Gain15/1 -> Sum11/1
  [Ics] -> Gain15/1
  [Vsumc] -> Gain16/1
  Sum12/1 -> Product5/1
  Sum9/1 -> Product4/1
  [Vsumb] -> Gain13/1
  [Ibs] -> Gain12/1
  Gain12/1 -> Sum10/1
  [Ibsum] -> Sum10/2
  [Vdiffb] -> Sum9/2
  Gain13/1 -> Sum9/1
  Integrator4/1 -> Divide4/2, [Vbls]
  Gain9/1 -> Integrator4/1
  Divide4/1 -> Gain9/1
  Product4/1 -> Divide4/1, Scope8/1
  Sum10/1 -> Product4/2
  Sum8/1 -> Product3/2
  Product3/1 -> Scope7/1, Divide3/1
  Divide3/1 -> Gain2/1
  Gain2/1 -> Integrator3/1
  Integrator3/1 -> [Vals], Divide3/2
  Gain11/1 -> Sum7/1
  [Vdiffa] -> Sum7/2
  [Iasum] -> Sum8/2
  Gain10/1 -> Sum8/1
  [Ias] -> Gain10/1
  [Vsuma] -> Gain11/1
  Sum7/1 -> Product3/1
  Sum5/1 -> Product2/1
  [Vsumc] -> Gain8/1
  [Ics] -> Gain7/1
  Gain7/1 -> Sum6/1
  [Icsum] -> Sum6/2
  [Vdiffc] -> Sum5/2
  Gain8/1 -> Sum5/1
  Integrator2/1 -> Divide2/2, [Vcus]
  Gain14/1 -> Integrator2/1
  Divide2/1 -> Gain14/1
  Product2/1 -> Divide2/1, Scope6/1
  Sum6/1 -> Product2/2
  Sum4/1 -> Product1/2
  Product1/1 -> Scope5/1, Divide1/1
  Divide1/1 -> Gain5/1
  Gain5/1 -> Integrator1/1
  Integrator1/1 -> [Vbus], Divide1/2
  Gain4/1 -> Sum3/1
  [Vdiffb] -> Sum3/2
  [Ibsum] -> Sum4/2
  Gain3/1 -> Sum4/1
  [Ibs] -> Gain3/1
  [Vsumb] -> Gain4/1
  Sum3/1 -> Product1/1
  Sum1/1 -> Product/1
  [Vsuma] -> Gain6/1
  [Ias] -> Gain1/1
  Gain1/1 -> Sum2/1
  [Iasum] -> Sum2/2
  [Vdiffa] -> Sum1/2
  Gain6/1 -> Sum1/1
  [Vsumc] -> Controlled Voltage Source6/1
  [Vsumb] -> Controlled Voltage Source5/1
  [Vsuma] -> Controlled Voltage Source4/1
  Mesura Ias12/1 -> [Icsum]
  Mesura Ias11/1 -> [Ibsum]
  Mesura Ias1/1 -> [Iasum]
  [Vdiffc] -> Scope14/3, Controlled Voltage Source3/1
  [Vdiffb] -> Scope14/2, Controlled Voltage Source2/1
  [Vdiffa] -> Scope14/1, Controlled Voltage Source1/1
  Integrator/1 -> Divide/2, [Vaus]
  Gain/1 -> Integrator/1
  Divide/1 -> Gain/1
  Product/1 -> Divide/1, Scope4/1
  Sum2/1 -> Product/2
  Mux3/1 -> Vs/1, Scope3/1
  [Vcls] -> Mux3/6  "Vcls"
  [Vcus] -> Mux3/5  "Vcus"
  [Vbls] -> Mux3/4  "Vbls"
  [Vbus] -> Mux3/3  "Vbus"
  [Vals] -> Mux3/2  "Vals"
  [Vaus] -> Mux3/1  "Vaus"
  [Icl] -> Mux2/3
  Mux2/1 -> Il/1, Scope2/1
  [Ial] -> Mux2/1
  Mux1/1 -> Iu/1, Scope1/1
  [Icu] -> Mux1/3
  [Ibu] -> Mux1/2
  [Iau] -> Mux1/1
  [Ias] -> Mux/1  "Ias"
  [Ibs] -> Mux/2  "Ibs"
  [Ics] -> Mux/3  "Ics"
  Mux/1 -> Is/1, Scope/1
  Demux/4 -> [Vsuma]
  Demux/2 -> [Vdiffb]
  Demux/3 -> [Vdiffc]
  Demux/1 -> [Vdiffa]
  Demux/6 -> [Vsumc]
  Demux/5 -> [Vsumb]
  Vdiff,sum/1 -> Scope10/1, Demux/1
  Mesura Ias9/1 -> [Ibs]
  Mesura Ias7/1 -> [Ias]
  Mesura Ias10/1 -> [Ics]
  [Iasum] -> Mux4/1
  [Iasum] -> Mux4/2
  [Iasum] -> Mux4/3
  Mux4/1 -> Scope11/1
  Current Measurement/1 -> Product6/1
  Voltage Measurement/1 -> Product6/2
  Product6/1 -> Display/1, Scope12/1
  Voltage Measurement1/1 -> Scope13/1
  connections:
  Mesura Ias12/RConn1 -- Mesura Ias11/RConn1 -- Mesura Ias1/RConn1 -- Voltage Measurement/LConn2 -- VDC-/RConn1
  Voltage Measurement/LConn1 -- Current Measurement/LConn1 -- Controlled Voltage Source6/RConn1 -- Controlled Voltage Source5/RConn1 -- Voltage Measurement1/LConn1 -- Controlled Voltage Source4/RConn1
  Controlled Voltage Source1/LConn1 -- Controlled Voltage Source3/LConn1 -- Controlled Voltage Source2/LConn1
  Controlled Voltage Source3/RConn1 -- Zsa2/LConn1
  Controlled Voltage Source2/RConn1 -- Zsa1/LConn1
  Controlled Voltage Source1/RConn1 -- Zsa/LConn1
  Zsa2/RConn1 -- Mesura Ias10/LConn1
  Zsa1/RConn1 -- Mesura Ias9/LConn1
  Zsa/RConn1 -- Mesura Ias7/LConn1
  Mesura Ias10/RConn1 -- VC/RConn1
  Mesura Ias9/RConn1 -- VB/RConn1
  Mesura Ias7/RConn1 -- VA/RConn1
  Zsa3/LConn1 -- Controlled Voltage Source4/LConn1 -- Voltage Measurement1/LConn2
  Zsa3/RConn1 -- Mesura Ias1/LConn1
  Zsa4/LConn1 -- Controlled Voltage Source5/LConn1
  Zsa4/RConn1 -- Mesura Ias11/LConn1
  Zsa5/LConn1 -- Controlled Voltage Source6/LConn1
  Zsa5/RConn1 -- Mesura Ias12/LConn1
  Current Measurement/RConn1 -- VDC+/RConn1

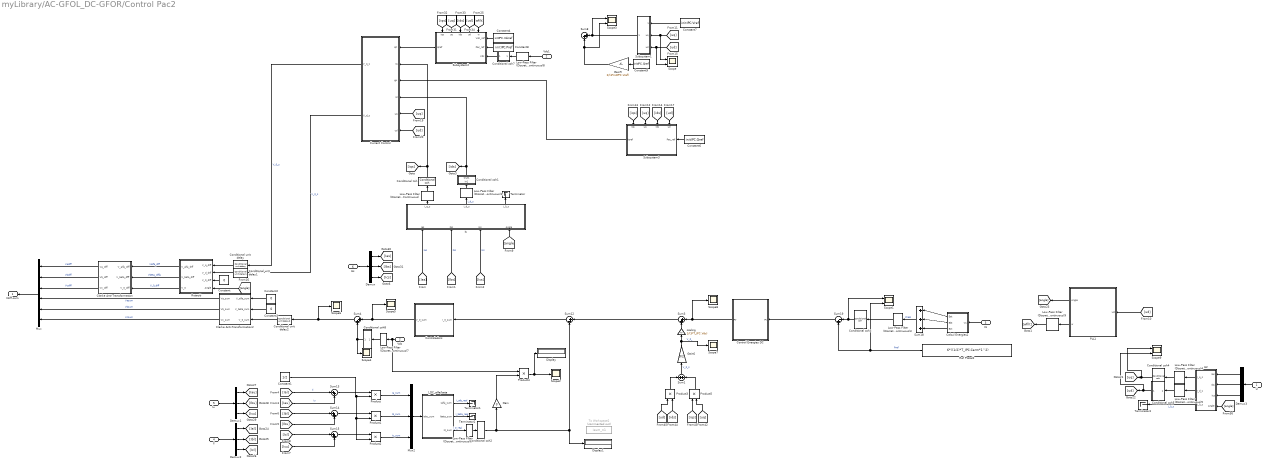
== system myLibrary/AC-GFOL_DC-GFOR/Control Pac2 ==
  U : Inport
  Vdc : Inport  Port=2
  Vs : Inport  Port=3
  Il : Inport  Port=4
  Iu : Inport  Port=5
  Iss : Inport  Port=6
  Calcul Energies2 : Subsystem
  Clarke Anti-Transformation : Subsystem
  Clarke Anti-Transformation2 : Subsystem
  Conditional unit delay : $bdroot/GFOL/Control/Conditional unit delay  SystemSampleTime=-1  VariantActivationTime=update diagram  AllowFlexibleInterface=on  Latency=0  AutoFrameSizeCalculation=off
      link override Constant4: Value=T_IPC.tau_cmd
      link override Unit Delay2: InitialCondition=initIPC.vdiffq  SampleTime=T_IPC.tau_cmd
  Conditional unit delay1 : $bdroot/AC-GFOL_DC-GFOL/Control Pac2/Conditional unit delay1  SystemSampleTime=-1  VariantActivationTime=update diagram  AllowFlexibleInterface=on  Latency=0  AutoFrameSizeCalculation=off
  Conditional unit delay2 : $bdroot/AC-GFOL_DC-GFOL/Control Pac2/Conditional unit delay2  SystemSampleTime=-1  VariantActivationTime=update diagram  AllowFlexibleInterface=on  Latency=0  AutoFrameSizeCalculation=off
  Conditional zoh{,2..4} (4 alike) : $bdroot/AC-GFOL_DC-GFOL/Control Pac2/Conditional zoh  SystemSampleTime=-1  VariantActivationTime=update diagram  AllowFlexibleInterface=on  Latency=0  AutoFrameSizeCalculation=off
  Conditional zoh1 : Subsystem
  Conditional zoh5 : Subsystem
  Conditional zoh7 : Subsystem
  Conditional zoh8 : Subsystem
  Constant : Constant  Value=0
  Constant1 : Constant  Value=1/2
  Constant2 : Constant  Value=0
  Constant3 : Constant  Value=0
  Constant4 : Constant  Value=initIPC.Vdcref
  Constant6 : Constant  Value=initIPC.Qref
  Constant7 : Constant  Value=initIPC.Vref
  Constant8 : Constant  Value=initIPC.Pref
  Constant9 : Constant  Value=initIPC.Qref
  Control Energies DC : Subsystem
  Controladors : Subsystem
  Current Control : Subsystem
  Demux{,1..3} (4 alike) : Demux  Outputs=3
  Display : Display
  Display1 : Display
  Gain : Gain  Gain=3
  Gain6 : Gain  Gain=3/2
  Gain9 : Gain  Gain=2/(3*initIPC.Vref)
  Is : Subsystem
  Is2 : Subsystem
  Low-Pass Filter (Discrete or Continuous) : eeGeneralControl/Low-Pass Filter (Discrete or Continuous)  K=1  T=T_IPC.delay  B=inf  A=-inf  init_option=Specify as parameter  x0=initIPC.idiffq  Ts=0
  Low-Pass Filter (Discrete or Continuous)1 : eeGeneralControl/Low-Pass Filter (Discrete or Continuous)  K=1  T=T_IPC.delay  B=inf  A=-inf  init_option=Specify as parameter  x0=initIPC.idiffd  Ts=0
  Low-Pass Filter (Discrete or Continuous)3 : eeGeneralControl/Low-Pass Filter (Discrete or Continuous)  K=1  T=T_IPC.delay  B=inf  A=-inf  init_option=Specify as parameter  x0=6*((1/2)*T_IPC.Carm*1^2)  Ts=0
  Low-Pass Filter (Discrete or Continuous)4 : eeGeneralControl/Low-Pass Filter (Discrete or Continuous)  K=1  T=T_IPC.delay  B=inf  A=-inf  init_option=Specify as parameter  x0=initIPC.uq  Ts=0
  Low-Pass Filter (Discrete or Continuous)5 : eeGeneralControl/Low-Pass Filter (Discrete or Continuous)  K=1  T=T_IPC.delay  B=inf  A=-inf  init_option=Specify as parameter  x0=initIPC.ud  Ts=0
  Low-Pass Filter (Discrete or Continuous)6 : eeGeneralControl/Low-Pass Filter (Discrete or Continuous)  K=1  T=T_IPC.delay  B=inf  A=-inf  init_option=Specify as parameter  x0=initIPC.isum0_DC  Ts=0
  Low-Pass Filter (Discrete or Continuous)7 : eeGeneralControl/Low-Pass Filter (Discrete or Continuous)  K=1  T=T_IPC.delay  B=inf  A=-inf  init_option=Specify as parameter  x0=initIPC.Vdc  Ts=0
  Low-Pass Filter (Discrete or Continuous)8 : eeGeneralControl/Low-Pass Filter (Discrete or Continuous)  K=1  T=T_IPC.delay  B=inf  A=-inf  init_option=Specify as parameter  x0=initIPC.Vdc  Ts=0
  Low-Pass Filter (Discrete or Continuous)9 : eeGeneralControl/Low-Pass Filter (Discrete or Continuous)  K=1  T=T_IPC.tw  B=inf  A=-inf  init_option=Specify as parameter  x0=2*pi*T_IPC.fb  Ts=0
  Mux : Mux  Inputs=6
  Mux2 : Mux  Inputs=3
  PLL1 : Subsystem
  Product{,1..5} (6 alike) : Product
  Ref Ptotal2 : Constant  Value=6*((1/2)*T_IPC.Carm*1^2)
  Rotació : Subsystem
  Scope{,1,3,9} (4 alike) : Scope  NumInputPorts=2
  Scope{2,4..8} (6 alike) : Scope
  Subsystem1 : Subsystem
      settings: PortSchema="{\"entries\":[{\"content\":{\"sides\":[{\"content\":{\"connectorIds\":[\"Out1\"]},\"type\":\"ConnectorPlacement.EquallySpacedRectSide\",\"uuid\":\"effe47ce-951a-4fb1-8fc1-e963775b8c82\"},{\"content\":{\"connectorIds\":[\"In1\",\"In2\",\"In3\"],\"side\":\"RIGHT\"},\"type\":\"ConnectorPlacement.EquallySpacedRectSide\",\"uuid\":\"a859b59d-6664-4e67-878a-4ecbefd8f8f0\"},{\"content\":{\"connectorIds\":[],\"side\":\"TOP\"},\"type\":\"ConnectorPlacement.EquallySpacedRectSide\",\"uuid\":\"0b762440-c8d9-40a7-a5db-13c46bc0406e\"}]},\"type\":\"ConnectorPlacement.EquallySpacedConnector\",\"uuid\":\"dbc4fef9-6b40-4568-97c6-19f27935f422\"}],\"packageUris\":[\"http://schema.mathworks.com/mf0/Connector/R2020b\"],\"version\":\"1.0\"}"
  Subsystem2 : Subsystem
      settings: PortSchema="{\"entries\":[{\"content\":{\"sides\":[{\"content\":{\"connectorIds\":[\"Out1\"]},\"type\":\"ConnectorPlacement.EquallySpacedRectSide\",\"uuid\":\"dea8424c-00e8-4bd8-a696-176e9d81b4b0\"},{\"content\":{\"connectorIds\":[\"In6\",\"In7\",\"In8\"],\"side\":\"RIGHT\"},\"type\":\"ConnectorPlacement.EquallySpacedRectSide\",\"uuid\":\"15b830a2-0897-480b-96a6-ff349e082a47\"},{\"content\":{\"connectorIds\":[\"In1\",\"In2\",\"In3\",\"In4\",\"In5\"],\"side\":\"TOP\"},\"type\":\"ConnectorPlacement.EquallySpacedRectSide\",\"uuid\":\"07916eec-e3fd-4ba3-9129-5b3a9aa06051\"}]},\"type\":\"ConnectorPlacement.EquallySpacedConnector\",\"uuid\":\"22000632-3c2a-414c-a4d7-471046f1c1a1\"}],\"packageUris\":[\"http://schema.mathworks.com/mf0/Connector/R2020b\"],\"version\":\"1.0\"}"
  Subsystem3 : Subsystem  AncestorBlock=myLibrary/AC-GFOL_DC-GFOR/Control Pac2/Subsystem2
      settings: PortSchema="{\"entries\":[{\"content\":{\"sides\":[{\"content\":{\"connectorIds\":[\"Out1\"]},\"type\":\"ConnectorPlacement.EquallySpacedRectSide\",\"uuid\":\"dea8424c-00e8-4bd8-a696-176e9d81b4b0\"},{\"content\":{\"connectorIds\":[\"In5\"],\"side\":\"RIGHT\"},\"type\":\"ConnectorPlacement.EquallySpacedRectSide\",\"uuid\":\"15b830a2-0897-480b-96a6-ff349e082a47\"},{\"content\":{\"connectorIds\":[\"In1\",\"In2\",\"In3\",\"In4\"],\"side\":\"TOP\"},\"type\":\"ConnectorPlacement.EquallySpacedRectSide\",\"uuid\":\"07916eec-e3fd-4ba3-9129-5b3a9aa06051\"}]},\"type\":\"ConnectorPlacement.EquallySpacedConnector\",\"uuid\":\"22000632-3c2a-414c-a4d7-471046f1c1a1\"}],\"packageUris\":[\"http://schema.mathworks.com/mf0/Connector/R2020b\"],\"version\":\"1.0\"}"
  Sum1 : Sum
  Sum12 : Sum  Inputs=|+-
  Sum{3..4,8,13..15} (6 alike) : Sum  Inputs=|++
  Sum18 : Sum  Inputs=|+++
  Sum19 : Sum  Inputs=|-+
  Terminator{,1..2,4} (4 alike) : Terminator
  To Workspace2 : ToWorkspace  Commented=on  VariableName=isum_n1  SampleTime=plots_step
  Vdc1 : InportShadow  Port=2
  l_DC_alfa/beta : Subsystem
  scaling : Gain  Gain=1/(3*T_IPC.Vdc)
  Vdiff-sum : Outport
  wires:
  Low-Pass Filter (Discrete or Continuous)9/1 -> [wfilt]
  PLL1/2(w) -> Low-Pass Filter (Discrete or Continuous)9/1
  Is/3(I_0_s) -> Terminator/1
  Low-Pass Filter (Discrete or Continuous)7/1 -> Conditional zoh8/1(In1)
  Low-Pass Filter (Discrete or Continuous)3/1 -> Conditional zoh3/1
  Low-Pass Filter (Discrete or Continuous)4/1 -> Conditional zoh4/1
  Low-Pass Filter (Discrete or Continuous)5/1 -> Conditional zoh5/1(In1)
  Low-Pass Filter (Discrete or Continuous)1/1 -> Conditional zoh1/1(In1)
  Low-Pass Filter (Discrete or Continuous)/1 -> Conditional zoh/1
  Ref Ptotal2/1 -> Scope1/2, Sum19/2  "Pref"
  Calcul Energies2/1(Eat) -> Sum18/1
  Constant2/1 -> Clarke Anti-Transformation2/1(V_alfa_sum)
  Constant3/1 -> Clarke Anti-Transformation2/2(V_beta_sum)
  Mux/1 -> Vdiff-sum/1
  Clarke Anti-Transformation2/1(Va_sum) -> Mux/4  "Vasum"
  Clarke Anti-Transformation2/2(Vb_sum) -> Mux/5  "Vbsum"
  Clarke Anti-Transformation/3(Vc_diff) -> Mux/3  "Vcdiff"
  Clarke Anti-Transformation/2(Vb_diff) -> Mux/2  "Vbdiff"
  Clarke Anti-Transformation/1(Va_diff) -> Mux/1  "Vadiff"
  Rotació/1(V_alfa_diff) -> Clarke Anti-Transformation/1(V_alfa_diff)  "Valfa_diff"
  Rotació/3(V_0) -> Clarke Anti-Transformation/3(V_0_diff)  "V_0_diff"
  [Ias] -> Is/1(Ias)  "Ias"
  [Ics] -> Is/3(Ics)  "Ics"
  [Ibs] -> Is/2(Ibs)  "Ibs"
  Rotació/2(V_beta_diff) -> Clarke Anti-Transformation/2(V_beta_dfff)  "Vbeta_diffa"
  Mux2/1 -> l_DC_alfa/beta/1(Iabc_sum)
  Product/1 -> Mux2/1  "Ia_sum"
  [Ial] -> Sum13/1  "Il"
  [Iau] -> Sum13/2  "Iu"
  Sum13/1 -> Product/1
  Constant1/1 -> Product2/2, Product1/2, Product/2
  Product1/1 -> Mux2/2  "Ib_sum"
  [Ibl] -> Sum14/1
  [Ibu] -> Sum14/2
  Sum14/1 -> Product1/1
  Product2/1 -> Mux2/3  "Ic_sum"
  [Icl] -> Sum15/1
  [Icu] -> Sum15/2
  Sum15/1 -> Product2/1
  Clarke Anti-Transformation2/3(Vc_sum) -> Mux/6  "Vcsum"
  Iu/1 -> Demux1/1
  Demux2/2 -> [Ibl]
  Demux1/1 -> [Iau]
  Demux1/3 -> [Icu]
  Il/1 -> Demux2/1
  Demux2/3 -> [Icl]
  Demux2/1 -> [Ial]
  Demux1/2 -> [Ibu]
  Demux3/2 -> Is2/2(Ibs)
  [angle] -> Is2/4(Angle)
  PLL1/1(Angle) -> [angle]
  [ud] -> PLL1/1(Ud)
  U/1 -> Demux3/1
  Demux3/3 -> Is2/3(Ics)
  Demux3/1 -> Is2/1(Ias)
  Demux/1 -> [Ias]
  Demux/2 -> [Ibs]
  Demux/3 -> [Ics]
  Iss/1 -> Demux/1
  Vs/1 -> Calcul Energies2/1(Vs)
  Calcul Energies2/3(Ect) -> Sum18/3
  Calcul Energies2/2(Ebt) -> Sum18/2
  [angle] -> Is/4(Angle)
  [angle] -> Rotació/4(Angle)
  Current Control/1(V_q_s) -> Conditional unit delay/1  "V_0_s"
  [uq] -> Current Control/5(uq)
  [ud] -> Current Control/6(ud)
  Controladors/1(V_0_sum) -> Scope5/1, Sum4/1
  Sum12/1 -> Controladors/1(I_0_sum)
  Sum19/1 -> Control Energies DC/1(Pt)
  Constant7/1 -> Subsystem1/1(uref)
  [uq] -> Scope/1, Subsystem1/2(uq)
  [ud] -> Scope/2, Subsystem1/3(ud)
  Sum4/1 -> Scope6/1, Conditional unit delay2/1
  Is2/3(I_0_s) -> Terminator4/1  "I_0_s"
  Subsystem2/1(iqref) -> Current Control/1(Iq*)
  [ud] -> Product3/1
  [uq] -> Product5/2
  Gain6/1 -> Scope7/1, scaling/1  "V_0_"
  Sum1/1 -> Gain6/1  "V_0_s"
  Product5/1 -> Sum1/2
  Control Energies DC/1(Pt') -> Scope8/1, Sum3/1
  [iqs] -> Product5/1
  scaling/1 -> Sum3/2
  Sum3/1 -> Sum12/1
  Product3/1 -> Sum1/1
  [ids] -> Product3/2
  Subsystem1/1(idref) -> Scope3/1, Sum8/1
  Constant9/1 -> Gain9/1
  Gain9/1 -> Scope3/2, Sum8/2
  Current Control/2(V_d_s) -> Conditional unit delay1/1  "V_0_s"
  Constant/1 -> Rotació/3(V_0_diff)
  l_DC_alfa/beta/1(Ialfa_sum) -> Terminator1/1  "I_afa_real"
  l_DC_alfa/beta/2(Ibeta_sum) -> Terminator2/1  "I_beta_real"
  Constant8/1 -> Subsystem2/7(Pac_ref)
  Vdc1/1 -> Low-Pass Filter (Discrete or Continuous)8/1
  Low-Pass Filter (Discrete or Continuous)8/1 -> Conditional zoh7/1(In1)
  Constant4/1 -> Subsystem2/6(Vdc_ref)
  [wfilt] -> Subsystem2/5(w)
  [ud] -> Subsystem2/4(ud)
  [ids] -> Subsystem2/3(ids)
  [uq] -> Subsystem2/2(uq)
  [iqs] -> Subsystem2/1(iqs)
  Gain/1 -> Product4/2
  Product4/1 -> Display/1, Scope2/1
  [uq] -> Subsystem3/2(uq)
  [ud] -> Subsystem3/4(ud)
  [ids] -> Subsystem3/3(ids)
  Constant6/1 -> Subsystem3/5(Pac_ref)
  [iqs] -> Subsystem3/1(iqs)
  Subsystem3/1(iqref) -> Current Control/3(Id*)
  Conditional unit delay1/1 -> Rotació/2(V_d_diff)
  Conditional unit delay/1 -> Rotació/1(V_q_diff)
  Vdc/1 -> Low-Pass Filter (Discrete or Continuous)7/1, Product4/1
  Conditional unit delay2/1 -> Clarke Anti-Transformation2/3(V_0_sum)
  Conditional zoh7/1(Out1) -> Subsystem2/8(Vdc)
  Conditional zoh8/1(Out1) -> Scope4/1, Sum4/2
  l_DC_alfa/beta/3(I0_sum) -> Low-Pass Filter (Discrete or Continuous)6/1  "I_0_real"
  Low-Pass Filter (Discrete or Continuous)6/1 -> Conditional zoh2/1
  Conditional zoh2/1 -> Gain/1, Sum12/2, Display1/1
  Sum18/1 -> Low-Pass Filter (Discrete or Continuous)3/1  "Preal"
  Conditional zoh3/1 -> Scope1/1, Sum19/1
  Is2/1(I_q_s) -> Low-Pass Filter (Discrete or Continuous)4/1
  Is2/2(I_d_s) -> Low-Pass Filter (Discrete or Continuous)5/1
  Conditional zoh5/1(Out1) -> Scope9/2, [ud]
  Conditional zoh4/1 -> Scope9/1, [uq]
  Is/1(I_q_s) -> Low-Pass Filter (Discrete or Continuous)/1
  Conditional zoh/1 -> Current Control/2(Iq), [iqs]
  Is/2(I_d_s) -> Low-Pass Filter (Discrete or Continuous)1/1  "I_d_s"
  Conditional zoh1/1(Out1) -> Current Control/4(Id), [ids]
